simulink model "Tracking"  (R2017a)
settings: Solver=VariableStepAuto  StartTime=0.0  StopTime=0.5  RelTol=1e-3
undefined symbols (not defined in the file): magnitude
libraries: commfilt2 x24, simulink x16, dspmtrx3 x12, dspswit3 x8
(part 2 of 2)

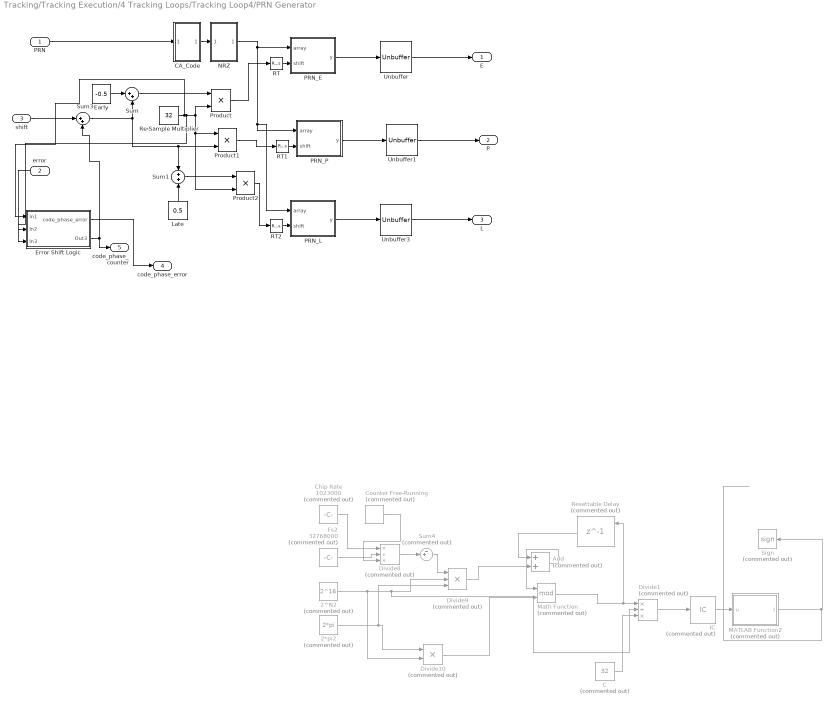
== system Tracking/Tracking Execution/4 Tracking Loops/Tracking Loop4/PRN Generator  ==
  PRN : Inport
  error : Inport  Port=2  SampleTime=0.001
  shift : Inport  Port=3
  2*pi2 : Constant  Commented=on  Value=2*pi
  2^N2 : Constant  Commented=on  Value=2^16
  Add : Sum  Commented=on
  C : Constant  Commented=on  Value=32
  "CA_Code " : Subsystem
  Chip Rate : Constant  Commented=on  Value=1023000
  Counter Free-Running : simulink/Sources/Counter Free-Running  Commented=on  NumBits=15  tsamp=1/32768000
  Divide1 : Product  Commented=on  Inputs=*/*
  Divide10 : Product  Commented=on
  Divide8 : Product  Commented=on  Inputs=*/*
  Divide9 : Product  Commented=on  Inputs=***
  Early : Constant  Value=-0.5
  Error Shift Logic : Subsystem
  Fs2 : Constant  Commented=on  Value=32768000
  IC : InitialCondition  Commented=on  Value=1023000
  Late : Constant  Value=0.5
  MATLAB Function2 : MATLAB Function  Commented=on  TreatAsAtomicUnit=on
  Math Function : Math  Commented=on  Operator=mod  SaturateOnIntegerOverflow=on
  NRZ : Subsystem
  PRN_E : MATLAB Function  TreatAsAtomicUnit=on  SystemSampleTime=0.001
  PRN_L : MATLAB Function  TreatAsAtomicUnit=on  SystemSampleTime=0.001
  PRN_P : MATLAB Function  TreatAsAtomicUnit=on  SystemSampleTime=0.001
  Product : Product
  Product1 : Product
  Product2 : Product
  RT : RateTransition  OutPortSampleTime=0.001
  RT1 : RateTransition  OutPortSampleTime=0.001
  RT2 : RateTransition  OutPortSampleTime=0.001
  Re-Sample Multiplier : Constant  Value=32
  Resettable Delay : Delay  Commented=on  DelayLength=1  ExternalReset=Rising  SampleTime=0.001
      settings: InputPortMap=u0,r5
  Sign : Signum  Commented=on
  Sum : Sum  Inputs=|++
  Sum1 : Sum
  Sum3 : Sum  Inputs=|++
  Sum4 : Sum  Commented=on  Inputs=-+|
  Unbuffer : Unbuffer
  Unbuffer1 : Unbuffer
  Unbuffer3 : Unbuffer
  E : Outport
  P : Outport  Port=2
  L : Outport  Port=3
  code_phase_error : Outport  Port=4
  code_phase_counter : Outport  Port=5
  wires:
  Product/1 -> RT/1
  PRN_E/1(y) -> Unbuffer/1
  Product2/1 -> RT2/1
  PRN_L/1(y) -> Unbuffer3/1
  Re-Sample Multiplier/1 -> Error Shift Logic/1(In1), Error Shift Logic/2(In2), Product1/1, Product2/2, Product/2
  PRN/1 -> "CA_Code "/1(In1)
  Unbuffer1/1 -> P/1
  Unbuffer3/1 -> L/1
  Early/1 -> Sum/1
  Sum/1 -> Product/1
  Sum3/1 -> Product1/2, Sum1/1, Sum/2
  Sum1/1 -> Product2/1
  PRN_P/1(y) -> Unbuffer1/1
  RT/1 -> PRN_E/2(shift)
  RT1/1 -> PRN_P/2(shift)
  RT2/1 -> PRN_L/2(shift)
  Late/1 -> Sum1/2
  "CA_Code "/1(Out1) -> NRZ/1(In1)
  Unbuffer/1 -> E/1
  NRZ/1(Out1) -> PRN_E/1(array), PRN_L/1(array), PRN_P/1(array)
  Product1/1 -> RT1/1
  MATLAB Function2/1(I) -> Sign/1
  Divide8/1 -> Sum4/2
  C/1 -> Divide1/3
  2^N2/1 -> Divide10/2, Divide1/2, Divide9/2
  Fs2/1 -> Divide8/2
  2*pi2/1 -> Divide9/3, Divide10/1
  Sum4/1 -> Divide9/1
  IC/1 -> MATLAB Function2/1(u)
  Divide10/1 -> Math Function/2
  Chip Rate/1 -> Divide8/1
  Resettable Delay/1 -> Add/1
  Divide1/1 -> IC/1
  Divide9/1 -> Add/2
  Counter Free-Running/1 -> Divide8/3
  Add/1 -> Math Function/1
  Math Function/1 -> Resettable Delay/1, Divide1/1
  shift/1 -> Sum3/1
  Error Shift Logic/2(Out3) -> code_phase_counter/1, Sum3/2
  error/1 -> Error Shift Logic/3(In3)
  Error Shift Logic/1(code_phase_error) -> code_phase_error/1

== system Tracking/Tracking Execution/4 Tracking Loops/Tracking Loop1/Carrier Filter/Subsystem ==
  BW : Constant  Value=50
  C1 : Subsystem
  C2 : Subsystem
  Constant1 : Constant  Value=8
  Constant2 : Constant  Value=4
  Constant4 : Constant
  Damping : Constant  Value=0.7
  K : Constant  Value=4
  T : Constant  Value=0.001
  Wn : Subsystem
  "K2 " : Outport
  K1 : Outport  Port=2
  wires:
  C1/1(Out1) -> K1/1
  Constant1/1 -> C1/1(In1), Wn/1(In1)
  BW/1 -> Wn/2(In2)
  Damping/1 -> C1/2(In2), C1/3(In3), Wn/3(In3), C2/3(In3), C2/2(In2)
  Constant2/1 -> C2/5(In5), C1/7(In7), C2/6(In6), C2/7(In7), C1/8(In8), Wn/4(In4)
  Constant4/1 -> Wn/5(In5)
  T/1 -> C1/4(In4), C1/5(In5), C1/6(In6), C2/4(In4)
  Wn/1(Out1) -> C1/10(In10), C2/8(In8), C1/9(In9)
  C2/1(Out1) -> "K2 "/1
  K/1 -> C1/11(In11), C2/1(In1)

== system Tracking/Tracking Execution/4 Tracking Loops/Tracking Loop1/PRN Generator /CA_Code  ==
  In1 : Inport
  CA_Code : MATLAB Function  TreatAsAtomicUnit=on  SystemSampleTime=0.001
  Constant1 : Constant  Value=32
  Constant2 : Constant
  MinMax : MinMax  Function=max  Inputs=2
  RT : RateTransition  OutPortSampleTime=0.001
  Reshape : Reshape  OutputDimensionality=Column vector (2-D)
  Out1 : Outport
  wires:
  In1/1 -> RT/1
  CA_Code/1(g) -> Reshape/1
  Constant1/1 -> CA_Code/2(fs)
  Reshape/1 -> Out1/1
  RT/1 -> MinMax/2
  MinMax/1 -> CA_Code/1(sv)
  Constant2/1 -> MinMax/1

== system Tracking/Tracking Execution/4 Tracking Loops/Tracking Loop1/PRN Generator /Error Shift Logic ==
  In1 : Inport
  In2 : Inport  Port=2
  In3 : Inport  Port=3
  Compare To Constant2 : simulink/Logic and Bit Operations/Compare To Constant  relop=>=  const=1  OutDataTypeStr=uint8
  Compare To Constant3 : simulink/Logic and Bit Operations/Compare To Constant  relop=<=  const=-1  OutDataTypeStr=uint8
  Counter : dspswit3/Counter  Direction=Up  CountEvent=Non-zero sample  CounterSize=User defined  MaxCount=2^16  InitialCount=0  Output=Count  HitValue=32  ResetInput=off  SamplesPerFrame=1  Ts=1  CntDtype=double  HitDtype=Logical
  Counter1 : dspswit3/Counter  Direction=Up  CountEvent=Non-zero sample  CounterSize=User defined  MaxCount=2^16  InitialCount=0  Output=Count  HitValue=32  ResetInput=on  SamplesPerFrame=1  Ts=1  CntDtype=double  HitDtype=Logical
  Divide : Product  Inputs=*/
  Product3 : Product
  RT3 : RateTransition  OutPortSampleTime=0.001
  RT4 : RateTransition  OutPortSampleTime=0.001
  Rounding Function : Rounding  Operator=round
  Sum2 : Sum  Inputs=-+
  Sum5 : Sum  Inputs=+-
  Sum6 : Sum  Inputs=+-
  Unit Delay : UnitDelay  SampleTime=0.001
  code_phase_error : Outport
  Out3 : Outport  Port=2
  wires:
  Sum2/1 -> Divide/1
  Counter1/1 -> Sum2/2
  In3/1 -> Product3/1
  Counter/1 -> Sum2/1
  Unit Delay/1 -> Sum6/2
  Sum6/1 -> Sum5/1, Rounding Function/1
  Rounding Function/1 -> Sum5/2, Compare To Constant3/1, Compare To Constant2/1
  Compare To Constant2/1 -> RT4/1
  Sum5/1 -> Unit Delay/1
  RT3/1 -> Counter1/1
  Compare To Constant3/1 -> RT3/1
  Divide/1 -> Out3/1, code_phase_error/1
  Product3/1 -> Sum6/1
  RT4/1 -> Counter/1
  In1/1 -> Divide/2
  In2/1 -> Product3/2

== system Tracking/Tracking Execution/4 Tracking Loops/Tracking Loop1/PRN Generator /NRZ ==
  In1 : Inport
  Constant5 : Constant  Value=2  SampleTime=-1
  Constant6 : Constant  Value=-1
  Product4 : Product
  Sum4 : Sum  Inputs=|++
  Out1 : Outport
  wires:
  Constant6/1 -> Sum4/1
  Sum4/1 -> Out1/1
  Product4/1 -> Sum4/2
  In1/1 -> Product4/2
  Constant5/1 -> Product4/1

== system Tracking/Tracking Execution/4 Tracking Loops/Tracking Loop2/Carrier Filter/Subsystem ==
  BW : Constant  Value=50
  C1 : Subsystem
  C2 : Subsystem
  Constant1 : Constant  Value=8
  Constant2 : Constant  Value=4
  Constant4 : Constant
  Damping : Constant  Value=0.7
  K : Constant  Value=4
  T : Constant  Value=0.001
  Wn : Subsystem
  "K2 " : Outport
  K1 : Outport  Port=2
  wires:
  C1/1(Out1) -> K1/1
  Constant1/1 -> C1/1(In1), Wn/1(In1)
  BW/1 -> Wn/2(In2)
  Damping/1 -> C1/2(In2), C1/3(In3), Wn/3(In3), C2/3(In3), C2/2(In2)
  Constant2/1 -> C2/5(In5), C1/7(In7), C2/6(In6), C2/7(In7), C1/8(In8), Wn/4(In4)
  Constant4/1 -> Wn/5(In5)
  T/1 -> C1/4(In4), C1/5(In5), C1/6(In6), C2/4(In4)
  Wn/1(Out1) -> C1/10(In10), C2/8(In8), C1/9(In9)
  C2/1(Out1) -> "K2 "/1
  K/1 -> C1/11(In11), C2/1(In1)

== system Tracking/Tracking Execution/4 Tracking Loops/Tracking Loop2/PRN Generator /CA_Code  ==
  In1 : Inport
  CA_Code : MATLAB Function  TreatAsAtomicUnit=on  SystemSampleTime=0.001
  Constant1 : Constant  Value=32
  Constant2 : Constant
  MinMax : MinMax  Function=max  Inputs=2
  RT : RateTransition  OutPortSampleTime=0.001
  Reshape : Reshape  OutputDimensionality=Column vector (2-D)
  Out1 : Outport
  wires:
  In1/1 -> RT/1
  CA_Code/1(g) -> Reshape/1
  Constant1/1 -> CA_Code/2(fs)
  Reshape/1 -> Out1/1
  RT/1 -> MinMax/2
  MinMax/1 -> CA_Code/1(sv)
  Constant2/1 -> MinMax/1

== system Tracking/Tracking Execution/4 Tracking Loops/Tracking Loop2/PRN Generator /Error Shift Logic ==
  In1 : Inport
  In2 : Inport  Port=2
  In3 : Inport  Port=3
  Compare To Constant2 : simulink/Logic and Bit Operations/Compare To Constant  relop=>=  const=1  OutDataTypeStr=uint8
  Compare To Constant3 : simulink/Logic and Bit Operations/Compare To Constant  relop=<=  const=-1  OutDataTypeStr=uint8
  Counter : dspswit3/Counter  Direction=Up  CountEvent=Non-zero sample  CounterSize=User defined  MaxCount=2^16  InitialCount=0  Output=Count  HitValue=32  ResetInput=off  SamplesPerFrame=1  Ts=1  CntDtype=double  HitDtype=Logical
  Counter1 : dspswit3/Counter  Direction=Up  CountEvent=Non-zero sample  CounterSize=User defined  MaxCount=2^16  InitialCount=0  Output=Count  HitValue=32  ResetInput=on  SamplesPerFrame=1  Ts=1  CntDtype=double  HitDtype=Logical
  Divide : Product  Inputs=*/
  Product3 : Product
  RT3 : RateTransition  OutPortSampleTime=0.001
  RT4 : RateTransition  OutPortSampleTime=0.001
  Rounding Function : Rounding  Operator=round
  Sum2 : Sum  Inputs=-+
  Sum5 : Sum  Inputs=+-
  Sum6 : Sum  Inputs=+-
  Unit Delay : UnitDelay  SampleTime=0.001
  code_phase_error : Outport
  Out3 : Outport  Port=2
  wires:
  Sum2/1 -> Divide/1
  Counter1/1 -> Sum2/2
  In3/1 -> Product3/1
  Counter/1 -> Sum2/1
  Unit Delay/1 -> Sum6/2
  Sum6/1 -> Sum5/1, Rounding Function/1
  Rounding Function/1 -> Sum5/2, Compare To Constant3/1, Compare To Constant2/1
  Compare To Constant2/1 -> RT4/1
  Sum5/1 -> Unit Delay/1
  RT3/1 -> Counter1/1
  Compare To Constant3/1 -> RT3/1
  Divide/1 -> Out3/1, code_phase_error/1
  Product3/1 -> Sum6/1
  RT4/1 -> Counter/1
  In1/1 -> Divide/2
  In2/1 -> Product3/2

== system Tracking/Tracking Execution/4 Tracking Loops/Tracking Loop2/PRN Generator /NRZ ==
  In1 : Inport
  Constant5 : Constant  Value=2  SampleTime=-1
  Constant6 : Constant  Value=-1
  Product4 : Product
  Sum4 : Sum  Inputs=|++
  Out1 : Outport
  wires:
  Constant6/1 -> Sum4/1
  Sum4/1 -> Out1/1
  Product4/1 -> Sum4/2
  In1/1 -> Product4/2
  Constant5/1 -> Product4/1

== system Tracking/Tracking Execution/4 Tracking Loops/Tracking Loop3/Carrier Filter/Subsystem ==
  BW : Constant  Value=50
  C1 : Subsystem
  C2 : Subsystem
  Constant1 : Constant  Value=8
  Constant2 : Constant  Value=4
  Constant4 : Constant
  Damping : Constant  Value=0.7
  K : Constant  Value=4
  T : Constant  Value=0.001
  Wn : Subsystem
  "K2 " : Outport
  K1 : Outport  Port=2
  wires:
  C1/1(Out1) -> K1/1
  Constant1/1 -> C1/1(In1), Wn/1(In1)
  BW/1 -> Wn/2(In2)
  Damping/1 -> C1/2(In2), C1/3(In3), Wn/3(In3), C2/3(In3), C2/2(In2)
  Constant2/1 -> C2/5(In5), C1/7(In7), C2/6(In6), C2/7(In7), C1/8(In8), Wn/4(In4)
  Constant4/1 -> Wn/5(In5)
  T/1 -> C1/4(In4), C1/5(In5), C1/6(In6), C2/4(In4)
  Wn/1(Out1) -> C1/10(In10), C2/8(In8), C1/9(In9)
  C2/1(Out1) -> "K2 "/1
  K/1 -> C1/11(In11), C2/1(In1)

== system Tracking/Tracking Execution/4 Tracking Loops/Tracking Loop3/PRN Generator /CA_Code  ==
  In1 : Inport
  CA_Code : MATLAB Function  TreatAsAtomicUnit=on  SystemSampleTime=0.001
  Constant1 : Constant  Value=32
  Constant2 : Constant
  MinMax : MinMax  Function=max  Inputs=2
  RT : RateTransition  OutPortSampleTime=0.001
  Reshape : Reshape  OutputDimensionality=Column vector (2-D)
  Out1 : Outport
  wires:
  In1/1 -> RT/1
  CA_Code/1(g) -> Reshape/1
  Constant1/1 -> CA_Code/2(fs)
  Reshape/1 -> Out1/1
  RT/1 -> MinMax/2
  MinMax/1 -> CA_Code/1(sv)
  Constant2/1 -> MinMax/1

== system Tracking/Tracking Execution/4 Tracking Loops/Tracking Loop3/PRN Generator /Error Shift Logic ==
  In1 : Inport
  In2 : Inport  Port=2
  In3 : Inport  Port=3
  Compare To Constant2 : simulink/Logic and Bit Operations/Compare To Constant  relop=>=  const=1  OutDataTypeStr=uint8
  Compare To Constant3 : simulink/Logic and Bit Operations/Compare To Constant  relop=<=  const=-1  OutDataTypeStr=uint8
  Counter : dspswit3/Counter  Direction=Up  CountEvent=Non-zero sample  CounterSize=User defined  MaxCount=2^16  InitialCount=0  Output=Count  HitValue=32  ResetInput=off  SamplesPerFrame=1  Ts=1  CntDtype=double  HitDtype=Logical
  Counter1 : dspswit3/Counter  Direction=Up  CountEvent=Non-zero sample  CounterSize=User defined  MaxCount=2^16  InitialCount=0  Output=Count  HitValue=32  ResetInput=on  SamplesPerFrame=1  Ts=1  CntDtype=double  HitDtype=Logical
  Divide : Product  Inputs=*/
  Product3 : Product
  RT3 : RateTransition  OutPortSampleTime=0.001
  RT4 : RateTransition  OutPortSampleTime=0.001
  Rounding Function : Rounding  Operator=round
  Sum2 : Sum  Inputs=-+
  Sum5 : Sum  Inputs=+-
  Sum6 : Sum  Inputs=+-
  Unit Delay : UnitDelay  SampleTime=0.001
  code_phase_error : Outport
  Out3 : Outport  Port=2
  wires:
  Sum2/1 -> Divide/1
  Counter1/1 -> Sum2/2
  In3/1 -> Product3/1
  Counter/1 -> Sum2/1
  Unit Delay/1 -> Sum6/2
  Sum6/1 -> Sum5/1, Rounding Function/1
  Rounding Function/1 -> Sum5/2, Compare To Constant3/1, Compare To Constant2/1
  Compare To Constant2/1 -> RT4/1
  Sum5/1 -> Unit Delay/1
  RT3/1 -> Counter1/1
  Compare To Constant3/1 -> RT3/1
  Divide/1 -> Out3/1, code_phase_error/1
  Product3/1 -> Sum6/1
  RT4/1 -> Counter/1
  In1/1 -> Divide/2
  In2/1 -> Product3/2

== system Tracking/Tracking Execution/4 Tracking Loops/Tracking Loop3/PRN Generator /NRZ ==
  In1 : Inport
  Constant5 : Constant  Value=2  SampleTime=-1
  Constant6 : Constant  Value=-1
  Product4 : Product
  Sum4 : Sum  Inputs=|++
  Out1 : Outport
  wires:
  Constant6/1 -> Sum4/1
  Sum4/1 -> Out1/1
  Product4/1 -> Sum4/2
  In1/1 -> Product4/2
  Constant5/1 -> Product4/1

== system Tracking/Tracking Execution/4 Tracking Loops/Tracking Loop4/Carrier Filter/Subsystem ==
  BW : Constant  Value=50
  C1 : Subsystem
  C2 : Subsystem
  Constant1 : Constant  Value=8
  Constant2 : Constant  Value=4
  Constant4 : Constant
  Damping : Constant  Value=0.7
  K : Constant  Value=4
  T : Constant  Value=0.001
  Wn : Subsystem
  "K2 " : Outport
  K1 : Outport  Port=2
  wires:
  C1/1(Out1) -> K1/1
  Constant1/1 -> C1/1(In1), Wn/1(In1)
  BW/1 -> Wn/2(In2)
  Damping/1 -> C1/2(In2), C1/3(In3), Wn/3(In3), C2/3(In3), C2/2(In2)
  Constant2/1 -> C2/5(In5), C1/7(In7), C2/6(In6), C2/7(In7), C1/8(In8), Wn/4(In4)
  Constant4/1 -> Wn/5(In5)
  T/1 -> C1/4(In4), C1/5(In5), C1/6(In6), C2/4(In4)
  Wn/1(Out1) -> C1/10(In10), C2/8(In8), C1/9(In9)
  C2/1(Out1) -> "K2 "/1
  K/1 -> C1/11(In11), C2/1(In1)

== system Tracking/Tracking Execution/4 Tracking Loops/Tracking Loop4/PRN Generator /CA_Code  ==
  In1 : Inport
  CA_Code : MATLAB Function  TreatAsAtomicUnit=on  SystemSampleTime=0.001
  Constant1 : Constant  Value=32
  Constant2 : Constant
  MinMax : MinMax  Function=max  Inputs=2
  RT : RateTransition  OutPortSampleTime=0.001
  Reshape : Reshape  OutputDimensionality=Column vector (2-D)
  Out1 : Outport
  wires:
  In1/1 -> RT/1
  CA_Code/1(g) -> Reshape/1
  Constant1/1 -> CA_Code/2(fs)
  Reshape/1 -> Out1/1
  RT/1 -> MinMax/2
  MinMax/1 -> CA_Code/1(sv)
  Constant2/1 -> MinMax/1

== system Tracking/Tracking Execution/4 Tracking Loops/Tracking Loop4/PRN Generator /Error Shift Logic ==
  In1 : Inport
  In2 : Inport  Port=2
  In3 : Inport  Port=3
  Compare To Constant2 : simulink/Logic and Bit Operations/Compare To Constant  relop=>=  const=1  OutDataTypeStr=uint8
  Compare To Constant3 : simulink/Logic and Bit Operations/Compare To Constant  relop=<=  const=-1  OutDataTypeStr=uint8
  Counter : dspswit3/Counter  Direction=Up  CountEvent=Non-zero sample  CounterSize=User defined  MaxCount=2^16  InitialCount=0  Output=Count  HitValue=32  ResetInput=off  SamplesPerFrame=1  Ts=1  CntDtype=double  HitDtype=Logical
  Counter1 : dspswit3/Counter  Direction=Up  CountEvent=Non-zero sample  CounterSize=User defined  MaxCount=2^16  InitialCount=0  Output=Count  HitValue=32  ResetInput=on  SamplesPerFrame=1  Ts=1  CntDtype=double  HitDtype=Logical
  Divide : Product  Inputs=*/
  Product3 : Product
  RT3 : RateTransition  OutPortSampleTime=0.001
  RT4 : RateTransition  OutPortSampleTime=0.001
  Rounding Function : Rounding  Operator=round
  Sum2 : Sum  Inputs=-+
  Sum5 : Sum  Inputs=+-
  Sum6 : Sum  Inputs=+-
  Unit Delay : UnitDelay  SampleTime=0.001
  code_phase_error : Outport
  Out3 : Outport  Port=2
  wires:
  Sum2/1 -> Divide/1
  Counter1/1 -> Sum2/2
  In3/1 -> Product3/1
  Counter/1 -> Sum2/1
  Unit Delay/1 -> Sum6/2
  Sum6/1 -> Sum5/1, Rounding Function/1
  Rounding Function/1 -> Sum5/2, Compare To Constant3/1, Compare To Constant2/1
  Compare To Constant2/1 -> RT4/1
  Sum5/1 -> Unit Delay/1
  RT3/1 -> Counter1/1
  Compare To Constant3/1 -> RT3/1
  Divide/1 -> Out3/1, code_phase_error/1
  Product3/1 -> Sum6/1
  RT4/1 -> Counter/1
  In1/1 -> Divide/2
  In2/1 -> Product3/2

== system Tracking/Tracking Execution/4 Tracking Loops/Tracking Loop4/PRN Generator /NRZ ==
  In1 : Inport
  Constant5 : Constant  Value=2  SampleTime=-1
  Constant6 : Constant  Value=-1
  Product4 : Product
  Sum4 : Sum  Inputs=|++
  Out1 : Outport
  wires:
  Constant6/1 -> Sum4/1
  Sum4/1 -> Out1/1
  Product4/1 -> Sum4/2
  In1/1 -> Product4/2
  Constant5/1 -> Product4/1

== system Tracking/Tracking Execution/4 Tracking Loops/Tracking Loop1/Carrier Filter/Subsystem/C1 ==
  In1 : Inport
  In2 : Inport  Port=2
  In3 : Inport  Port=3
  In4 : Inport  Port=4
  In5 : Inport  Port=5
  In6 : Inport  Port=6
  In7 : Inport  Port=7
  In8 : Inport  Port=8
  In9 : Inport  Port=9
  In10 : Inport  Port=10
  In11 : Inport  Port=11
  Add1 : Sum  Inputs=+++
  Gain 3 : Product  Inputs=***/
  Gain 4 : Product  Inputs=***
  Math Function3 : Math  Operator=square  SaturateOnIntegerOverflow=on
  Product3 : Product
  Product4 : Product  Inputs=4
  Out1 : Outport
  wires:
  In5/1 -> Product4/4
  In7/1 -> Add1/3
  Gain 3/1 -> Out1/1
  In9/1 -> Product4/3
  In4/1 -> Product3/1
  In8/1 -> Product4/1
  In2/1 -> Gain 4/1
  In11/1 -> Gain 3/1
  In10/1 -> Product3/2, Gain 4/2
  In1/1 -> Gain 3/3
  In6/1 -> Gain 4/3
  In3/1 -> Product4/2
  Add1/1 -> Gain 3/4
  Product4/1 -> Add1/2
  Gain 4/1 -> Gain 3/2
  Math Function3/1 -> Add1/1
  Product3/1 -> Math Function3/1

== system Tracking/Tracking Execution/4 Tracking Loops/Tracking Loop1/Carrier Filter/Subsystem/C2 ==
  In1 : Inport
  In2 : Inport  Port=2
  In3 : Inport  Port=3
  In4 : Inport  Port=4
  In5 : Inport  Port=5
  In6 : Inport  Port=6
  In7 : Inport  Port=7
  In8 : Inport  Port=8
  Add : Sum  Inputs=+++
  Gain 1 : Product  Inputs=***/
  Gain 2 : Product  Inputs=***
  Math Function : Math  Operator=square  SaturateOnIntegerOverflow=on
  Math Function1 : Math  Operator=square  SaturateOnIntegerOverflow=on
  Product1 : Product
  Product2 : Product  Inputs=4
  Out1 : Outport
  wires:
  Product1/1 -> Math Function1/1
  Math Function1/1 -> Add/1
  Add/1 -> Gain 1/4
  In2/1 -> Gain 2/1
  In5/1 -> Add/3
  In7/1 -> Product2/1
  In3/1 -> Product2/2
  In1/1 -> Gain 1/3
  In6/1 -> Gain 1/2
  Product2/1 -> Add/2
  Gain 1/1 -> Out1/1
  Math Function/1 -> Gain 1/1
  In8/1 -> Product1/1, Gain 2/2, Product2/3
  In4/1 -> Product1/2, Product2/4, Gain 2/3
  Gain 2/1 -> Math Function/1

== system Tracking/Tracking Execution/4 Tracking Loops/Tracking Loop1/Carrier Filter/Subsystem/Wn ==
  In1 : Inport
  In2 : Inport  Port=2
  In3 : Inport  Port=3
  In4 : Inport  Port=4
  In5 : Inport  Port=5
  Add : Sum
  Divide1 : Product  Inputs=***/
  Math Function : Math  Operator=square  SaturateOnIntegerOverflow=on
  Wn1 : Product
  Out1 : Outport
  wires:
  In4/1 -> Wn1/2
  Add/1 -> Divide1/4
  Wn1/1 -> Add/1
  In3/1 -> Divide1/3, Math Function/1
  In2/1 -> Divide1/2
  Math Function/1 -> Wn1/1
  Divide1/1 -> Out1/1
  In1/1 -> Divide1/1
  In5/1 -> Add/2

== system Tracking/Tracking Execution/4 Tracking Loops/Tracking Loop2/Carrier Filter/Subsystem/C1 ==
  In1 : Inport
  In2 : Inport  Port=2
  In3 : Inport  Port=3
  In4 : Inport  Port=4
  In5 : Inport  Port=5
  In6 : Inport  Port=6
  In7 : Inport  Port=7
  In8 : Inport  Port=8
  In9 : Inport  Port=9
  In10 : Inport  Port=10
  In11 : Inport  Port=11
  Add1 : Sum  Inputs=+++
  Gain 3 : Product  Inputs=***/
  Gain 4 : Product  Inputs=***
  Math Function3 : Math  Operator=square  SaturateOnIntegerOverflow=on
  Product3 : Product
  Product4 : Product  Inputs=4
  Out1 : Outport
  wires:
  In5/1 -> Product4/4
  In7/1 -> Add1/3
  Gain 3/1 -> Out1/1
  In9/1 -> Product4/3
  In4/1 -> Product3/1
  In8/1 -> Product4/1
  In2/1 -> Gain 4/1
  In11/1 -> Gain 3/1
  In10/1 -> Product3/2, Gain 4/2
  In1/1 -> Gain 3/3
  In6/1 -> Gain 4/3
  In3/1 -> Product4/2
  Add1/1 -> Gain 3/4
  Product4/1 -> Add1/2
  Gain 4/1 -> Gain 3/2
  Math Function3/1 -> Add1/1
  Product3/1 -> Math Function3/1

== system Tracking/Tracking Execution/4 Tracking Loops/Tracking Loop2/Carrier Filter/Subsystem/C2 ==
  In1 : Inport
  In2 : Inport  Port=2
  In3 : Inport  Port=3
  In4 : Inport  Port=4
  In5 : Inport  Port=5
  In6 : Inport  Port=6
  In7 : Inport  Port=7
  In8 : Inport  Port=8
  Add : Sum  Inputs=+++
  Gain 1 : Product  Inputs=***/
  Gain 2 : Product  Inputs=***
  Math Function : Math  Operator=square  SaturateOnIntegerOverflow=on
  Math Function1 : Math  Operator=square  SaturateOnIntegerOverflow=on
  Product1 : Product
  Product2 : Product  Inputs=4
  Out1 : Outport
  wires:
  Product1/1 -> Math Function1/1
  Math Function1/1 -> Add/1
  Add/1 -> Gain 1/4
  In2/1 -> Gain 2/1
  In5/1 -> Add/3
  In7/1 -> Product2/1
  In3/1 -> Product2/2
  In1/1 -> Gain 1/3
  In6/1 -> Gain 1/2
  Product2/1 -> Add/2
  Gain 1/1 -> Out1/1
  Math Function/1 -> Gain 1/1
  In8/1 -> Product1/1, Gain 2/2, Product2/3
  In4/1 -> Product1/2, Product2/4, Gain 2/3
  Gain 2/1 -> Math Function/1

== system Tracking/Tracking Execution/4 Tracking Loops/Tracking Loop2/Carrier Filter/Subsystem/Wn ==
  In1 : Inport
  In2 : Inport  Port=2
  In3 : Inport  Port=3
  In4 : Inport  Port=4
  In5 : Inport  Port=5
  Add : Sum
  Divide1 : Product  Inputs=***/
  Math Function : Math  Operator=square  SaturateOnIntegerOverflow=on
  Wn1 : Product
  Out1 : Outport
  wires:
  In4/1 -> Wn1/2
  Add/1 -> Divide1/4
  Wn1/1 -> Add/1
  In3/1 -> Divide1/3, Math Function/1
  In2/1 -> Divide1/2
  Math Function/1 -> Wn1/1
  Divide1/1 -> Out1/1
  In1/1 -> Divide1/1
  In5/1 -> Add/2

== system Tracking/Tracking Execution/4 Tracking Loops/Tracking Loop3/Carrier Filter/Subsystem/C1 ==
  In1 : Inport
  In2 : Inport  Port=2
  In3 : Inport  Port=3
  In4 : Inport  Port=4
  In5 : Inport  Port=5
  In6 : Inport  Port=6
  In7 : Inport  Port=7
  In8 : Inport  Port=8
  In9 : Inport  Port=9
  In10 : Inport  Port=10
  In11 : Inport  Port=11
  Add1 : Sum  Inputs=+++
  Gain 3 : Product  Inputs=***/
  Gain 4 : Product  Inputs=***
  Math Function3 : Math  Operator=square  SaturateOnIntegerOverflow=on
  Product3 : Product
  Product4 : Product  Inputs=4
  Out1 : Outport
  wires:
  In5/1 -> Product4/4
  In7/1 -> Add1/3
  Gain 3/1 -> Out1/1
  In9/1 -> Product4/3
  In4/1 -> Product3/1
  In8/1 -> Product4/1
  In2/1 -> Gain 4/1
  In11/1 -> Gain 3/1
  In10/1 -> Product3/2, Gain 4/2
  In1/1 -> Gain 3/3
  In6/1 -> Gain 4/3
  In3/1 -> Product4/2
  Add1/1 -> Gain 3/4
  Product4/1 -> Add1/2
  Gain 4/1 -> Gain 3/2
  Math Function3/1 -> Add1/1
  Product3/1 -> Math Function3/1

== system Tracking/Tracking Execution/4 Tracking Loops/Tracking Loop3/Carrier Filter/Subsystem/C2 ==
  In1 : Inport
  In2 : Inport  Port=2
  In3 : Inport  Port=3
  In4 : Inport  Port=4
  In5 : Inport  Port=5
  In6 : Inport  Port=6
  In7 : Inport  Port=7
  In8 : Inport  Port=8
  Add : Sum  Inputs=+++
  Gain 1 : Product  Inputs=***/
  Gain 2 : Product  Inputs=***
  Math Function : Math  Operator=square  SaturateOnIntegerOverflow=on
  Math Function1 : Math  Operator=square  SaturateOnIntegerOverflow=on
  Product1 : Product
  Product2 : Product  Inputs=4
  Out1 : Outport
  wires:
  Product1/1 -> Math Function1/1
  Math Function1/1 -> Add/1
  Add/1 -> Gain 1/4
  In2/1 -> Gain 2/1
  In5/1 -> Add/3
  In7/1 -> Product2/1
  In3/1 -> Product2/2
  In1/1 -> Gain 1/3
  In6/1 -> Gain 1/2
  Product2/1 -> Add/2
  Gain 1/1 -> Out1/1
  Math Function/1 -> Gain 1/1
  In8/1 -> Product1/1, Gain 2/2, Product2/3
  In4/1 -> Product1/2, Product2/4, Gain 2/3
  Gain 2/1 -> Math Function/1

== system Tracking/Tracking Execution/4 Tracking Loops/Tracking Loop3/Carrier Filter/Subsystem/Wn ==
  In1 : Inport
  In2 : Inport  Port=2
  In3 : Inport  Port=3
  In4 : Inport  Port=4
  In5 : Inport  Port=5
  Add : Sum
  Divide1 : Product  Inputs=***/
  Math Function : Math  Operator=square  SaturateOnIntegerOverflow=on
  Wn1 : Product
  Out1 : Outport
  wires:
  In4/1 -> Wn1/2
  Add/1 -> Divide1/4
  Wn1/1 -> Add/1
  In3/1 -> Divide1/3, Math Function/1
  In2/1 -> Divide1/2
  Math Function/1 -> Wn1/1
  Divide1/1 -> Out1/1
  In1/1 -> Divide1/1
  In5/1 -> Add/2

== system Tracking/Tracking Execution/4 Tracking Loops/Tracking Loop4/Carrier Filter/Subsystem/C1 ==
  In1 : Inport
  In2 : Inport  Port=2
  In3 : Inport  Port=3
  In4 : Inport  Port=4
  In5 : Inport  Port=5
  In6 : Inport  Port=6
  In7 : Inport  Port=7
  In8 : Inport  Port=8
  In9 : Inport  Port=9
  In10 : Inport  Port=10
  In11 : Inport  Port=11
  Add1 : Sum  Inputs=+++
  Gain 3 : Product  Inputs=***/
  Gain 4 : Product  Inputs=***
  Math Function3 : Math  Operator=square  SaturateOnIntegerOverflow=on
  Product3 : Product
  Product4 : Product  Inputs=4
  Out1 : Outport
  wires:
  In5/1 -> Product4/4
  In7/1 -> Add1/3
  Gain 3/1 -> Out1/1
  In9/1 -> Product4/3
  In4/1 -> Product3/1
  In8/1 -> Product4/1
  In2/1 -> Gain 4/1
  In11/1 -> Gain 3/1
  In10/1 -> Product3/2, Gain 4/2
  In1/1 -> Gain 3/3
  In6/1 -> Gain 4/3
  In3/1 -> Product4/2
  Add1/1 -> Gain 3/4
  Product4/1 -> Add1/2
  Gain 4/1 -> Gain 3/2
  Math Function3/1 -> Add1/1
  Product3/1 -> Math Function3/1

== system Tracking/Tracking Execution/4 Tracking Loops/Tracking Loop4/Carrier Filter/Subsystem/C2 ==
  In1 : Inport
  In2 : Inport  Port=2
  In3 : Inport  Port=3
  In4 : Inport  Port=4
  In5 : Inport  Port=5
  In6 : Inport  Port=6
  In7 : Inport  Port=7
  In8 : Inport  Port=8
  Add : Sum  Inputs=+++
  Gain 1 : Product  Inputs=***/
  Gain 2 : Product  Inputs=***
  Math Function : Math  Operator=square  SaturateOnIntegerOverflow=on
  Math Function1 : Math  Operator=square  SaturateOnIntegerOverflow=on
  Product1 : Product
  Product2 : Product  Inputs=4
  Out1 : Outport
  wires:
  Product1/1 -> Math Function1/1
  Math Function1/1 -> Add/1
  Add/1 -> Gain 1/4
  In2/1 -> Gain 2/1
  In5/1 -> Add/3
  In7/1 -> Product2/1
  In3/1 -> Product2/2
  In1/1 -> Gain 1/3
  In6/1 -> Gain 1/2
  Product2/1 -> Add/2
  Gain 1/1 -> Out1/1
  Math Function/1 -> Gain 1/1
  In8/1 -> Product1/1, Gain 2/2, Product2/3
  In4/1 -> Product1/2, Product2/4, Gain 2/3
  Gain 2/1 -> Math Function/1

== system Tracking/Tracking Execution/4 Tracking Loops/Tracking Loop4/Carrier Filter/Subsystem/Wn ==
  In1 : Inport
  In2 : Inport  Port=2
  In3 : Inport  Port=3
  In4 : Inport  Port=4
  In5 : Inport  Port=5
  Add : Sum
  Divide1 : Product  Inputs=***/
  Math Function : Math  Operator=square  SaturateOnIntegerOverflow=on
  Wn1 : Product
  Out1 : Outport
  wires:
  In4/1 -> Wn1/2
  Add/1 -> Divide1/4
  Wn1/1 -> Add/1
  In3/1 -> Divide1/3, Math Function/1
  In2/1 -> Divide1/2
  Math Function/1 -> Wn1/1
  Divide1/1 -> Out1/1
  In1/1 -> Divide1/1
  In5/1 -> Add/2

== matlab function Tracking/Tracking Execution/4 Tracking Loops/Tracking Loop1/PRN Generator /CA_Code /CA_Code ==
  data: sv input; g output; fs input
function g=CAcode(sv,fs)
coder.extrinsic('warning')
% function G=CACODE(SV,FS) 
% Generates 1023 length C/A Codes for GPS PRNs 1-37
%
% 
% g: nx1023 matrix- with each PRN in each row with symbols 1 and 0
% sv: a row or column vector of the SV's to be generated
% 	 valid entries are 1 to 37
% fs: optional number of samples per chip (defaults to 1), fractional samples allowed, must be 1 or greater.
%
% For multiple samples per chip, function is a zero order hold. 
%
%
% For example to generate the C/A codes for PRN 6 and PRN 12 use:
% g=cacode([6 12]),
% and to generate the C/A codes for PRN 6 and PRN 12 at 5 MHz use
% g=cacode([6 12],5/1.023)
% 
%
% For more information refer to the "GPS SPS Signal Specification"
% http://www.navcen.uscg.gov/pubs/gps/sigspec/default.htm
%
% Dan Boschen 12-30-2007
% boschen@loglin.com

% Revision History
% rev 1.0 Dan Boschen 4-15-2007  Initial Release
%
% rev 1.1 Dan Boschen 7-15-2007  Corrected error with taps for PRN30, should be [2,7] was 
% 					incorrect as [1 7]. Thank you Jadah Zak for finding this.
%
%
% rev 1.2 Dan Boschen 12-26-2007 Fixed column index error when ceil ~ L 
%				Thank you Jared Meadows for finding this.
%
% rev 1.3 Dan Boschen 12-30-2007 Changed comment "first order hold" to
% "zero order hold".
%
% rev 1.4 Dan Boschen 6-1-2010   Updated email address in comments



if nargin<2
	fs=1;
end


if (max(sv)>37) || (min(sv)<1) || (min(size(sv))~=1)
	error('sv must be a row or column vector with integers between 1 and 37\n')
end

if fs<1
	error('fs must be 1 or greater\n')
end	

% force integers
testint=round(sv)-sv;
if testint ~= 0 
	warning('non-integer value entered for sv, rounding to closest integer\n');
	sv = round(sv);
end


% table of C/A Code Tap Selection (sets delay for G2 generator)
tap=[2 6;
    3 7;
    4 8;
    5 9;
    1 9;
    2 10;
    1 8;
    2 9;
    3 10;
    2 3;
    3 4;
    5 6;
    6 7;
    7 8;
    8 9;
    9 10;
    1 4;
    2 5;
    3 6;
    4 7;
    5 8;
    6 9;
    1 3;
    4 6;
    5 7;
    6 8;
    7 9;
    8 10;
    1 6;
    2 7;
    3 8;
    4 9
    5 10
    4 10
    1 7
    2 8
    4 10];

% G1 LFSR: x^10+x^3+1
s=[0 0 1 0 0 0 0 0 0 1];
n=length(s);
g1=ones(1,n);	%initialization vector for G1

%g=ones(1,38192);
%g2=ones(1,38192);
%gfs=ones(1,38192);

g=ones(1,65536/2);
g2=ones(1,65536/2);
gfs=ones(1,65536/2);

L=2^n-1;

% G2j LFSR: x^10+x^9+x^8+x^6+x^3+x^2+1
t=[0 1 1 0 0 1 0 1 1 1];
q=ones(1,n);	%initialization vector for G2

% generate C/A Code sequences:
tap_sel=tap(sv,:);
for inc=1:L
    g2(:,inc)=mod(sum(q(tap_sel),2),2);
    g(:,inc)=mod(g1(n)+g2(:,inc),2);
   g1=[mod(sum(g1.*s),2) g1(1:n-1)];
   q=[mod(sum(q.*t),2) q(1:n-1)];
end

%upsample to desired rate
if fs~=1
	%fractional upsampling with zero order hold
	index=0;
	for cnt = 1/fs:1/fs:L
		index=index+1;
		if ceil(cnt) > L   %traps a floating point error in index
			gfs(:,index)=g(:,L);
		else
			gfs(:,index)=g(:,ceil(cnt));
		end
	end 
	g=gfs;
end

== matlab function Tracking/MATLAB Function ==
  data: y output
function y = fcn()

%FORMAT: [SATELLITE #1 Parameters, ... ,SATELLITE #4 parameters]
%y =[0 (SV#) (frequency) (code phase);... ; 0 (SV#) (frequency) (code phase);]  
y = [0 1 9207000 0; 0 2 9207000 100;0 3 9207000 512;0 4 9207000 800];

== matlab function Tracking/Tracking Execution/4 Tracking Loops/Tracking Loop1/Oscillator/MATLAB Function2 ==
  data: u input; I output; Q output
function [I,Q]= fcn(u)

I = cos(u);
Q = sin(u);

== matlab function Tracking/Tracking Execution/4 Tracking Loops/Tracking Loop1/PRN Generator /MATLAB Function2 ==
  data: u input; I output
function I = fcn(u)

I = cos(u);

== matlab function Tracking/Tracking Execution/4 Tracking Loops/Tracking Loop1/PRN Generator /PRN_E ==
  data: array input; y output; shift input
function y = fcn(array, shift)

y = circshift(array, shift);

== matlab function Tracking/Tracking Execution/4 Tracking Loops/Tracking Loop1/PRN Generator /PRN_L ==
  data: array input; y output; shift input
function y = fcn(array, shift)

y = circshift(array, shift);

== matlab function Tracking/Tracking Execution/4 Tracking Loops/Tracking Loop2/Oscillator/MATLAB Function2 ==
  data: u input; I output; Q output
function [I,Q]= fcn(u)

I = cos(u);
Q = sin(u);

== matlab function Tracking/Tracking Execution/4 Tracking Loops/Tracking Loop2/PRN Generator /CA_Code /CA_Code ==
  data: sv input; g output; fs input
function g=CAcode(sv,fs)
coder.extrinsic('warning')
% function G=CACODE(SV,FS) 
% Generates 1023 length C/A Codes for GPS PRNs 1-37
%
% 
% g: nx1023 matrix- with each PRN in each row with symbols 1 and 0
% sv: a row or column vector of the SV's to be generated
% 	 valid entries are 1 to 37
% fs: optional number of samples per chip (defaults to 1), fractional samples allowed, must be 1 or greater.
%
% For multiple samples per chip, function is a zero order hold. 
%
%
% For example to generate the C/A codes for PRN 6 and PRN 12 use:
% g=cacode([6 12]),
% and to generate the C/A codes for PRN 6 and PRN 12 at 5 MHz use
% g=cacode([6 12],5/1.023)
% 
%
% For more information refer to the "GPS SPS Signal Specification"
% http://www.navcen.uscg.gov/pubs/gps/sigspec/default.htm
%
% Dan Boschen 12-30-2007
% boschen@loglin.com

% Revision History
% rev 1.0 Dan Boschen 4-15-2007  Initial Release
%
% rev 1.1 Dan Boschen 7-15-2007  Corrected error with taps for PRN30, should be [2,7] was 
% 					incorrect as [1 7]. Thank you Jadah Zak for finding this.
%
%
% rev 1.2 Dan Boschen 12-26-2007 Fixed column index error when ceil ~ L 
%				Thank you Jared Meadows for finding this.
%
% rev 1.3 Dan Boschen 12-30-2007 Changed comment "first order hold" to
% "zero order hold".
%
% rev 1.4 Dan Boschen 6-1-2010   Updated email address in comments



if nargin<2
	fs=1;
end


if (max(sv)>37) || (min(sv)<1) || (min(size(sv))~=1)
	error('sv must be a row or column vector with integers between 1 and 37\n')
end

if fs<1
	error('fs must be 1 or greater\n')
end	

% force integers
testint=round(sv)-sv;
if testint ~= 0 
	warning('non-integer value entered for sv, rounding to closest integer\n');
	sv = round(sv);
end


% table of C/A Code Tap Selection (sets delay for G2 generator)
tap=[2 6;
    3 7;
    4 8;
    5 9;
    1 9;
    2 10;
    1 8;
    2 9;
    3 10;
    2 3;
    3 4;
    5 6;
    6 7;
    7 8;
    8 9;
    9 10;
    1 4;
    2 5;
    3 6;
    4 7;
    5 8;
    6 9;
    1 3;
    4 6;
    5 7;
    6 8;
    7 9;
    8 10;
    1 6;
    2 7;
    3 8;
    4 9
    5 10
    4 10
    1 7
    2 8
    4 10];

% G1 LFSR: x^10+x^3+1
s=[0 0 1 0 0 0 0 0 0 1];
n=length(s);
g1=ones(1,n);	%initialization vector for G1

%g=ones(1,38192);
%g2=ones(1,38192);
%gfs=ones(1,38192);

g=ones(1,65536/2);
g2=ones(1,65536/2);
gfs=ones(1,65536/2);

L=2^n-1;

% G2j LFSR: x^10+x^9+x^8+x^6+x^3+x^2+1
t=[0 1 1 0 0 1 0 1 1 1];
q=ones(1,n);	%initialization vector for G2

% generate C/A Code sequences:
tap_sel=tap(sv,:);
for inc=1:L
    g2(:,inc)=mod(sum(q(tap_sel),2),2);
    g(:,inc)=mod(g1(n)+g2(:,inc),2);
   g1=[mod(sum(g1.*s),2) g1(1:n-1)];
   q=[mod(sum(q.*t),2) q(1:n-1)];
end

%upsample to desired rate
if fs~=1
	%fractional upsampling with zero order hold
	index=0;
	for cnt = 1/fs:1/fs:L
		index=index+1;
		if ceil(cnt) > L   %traps a floating point error in index
			gfs(:,index)=g(:,L);
		else
			gfs(:,index)=g(:,ceil(cnt));
		end
	end 
	g=gfs;
end

== matlab function Tracking/Tracking Execution/4 Tracking Loops/Tracking Loop2/PRN Generator /MATLAB Function2 ==
  data: u input; I output
function I = fcn(u)

I = cos(u);

== matlab function Tracking/Tracking Execution/4 Tracking Loops/Tracking Loop2/PRN Generator /PRN_E ==
  data: array input; y output; shift input
function y = fcn(array, shift)

y = circshift(array, shift);

== matlab function Tracking/Tracking Execution/4 Tracking Loops/Tracking Loop1/PRN Generator /PRN_P ==
  data: array input; y output size=32768; shift input
function y = fcn(array, shift)

y = circshift(array, shift);

== matlab function Tracking/Tracking Execution/4 Tracking Loops/Tracking Loop3/PRN Generator /CA_Code /CA_Code ==
  data: sv input; g output; fs input
function g=CAcode(sv,fs)
coder.extrinsic('warning')
% function G=CACODE(SV,FS) 
% Generates 1023 length C/A Codes for GPS PRNs 1-37
%
% 
% g: nx1023 matrix- with each PRN in each row with symbols 1 and 0
% sv: a row or column vector of the SV's to be generated
% 	 valid entries are 1 to 37
% fs: optional number of samples per chip (defaults to 1), fractional samples allowed, must be 1 or greater.
%
% For multiple samples per chip, function is a zero order hold. 
%
%
% For example to generate the C/A codes for PRN 6 and PRN 12 use:
% g=cacode([6 12]),
% and to generate the C/A codes for PRN 6 and PRN 12 at 5 MHz use
% g=cacode([6 12],5/1.023)
% 
%
% For more information refer to the "GPS SPS Signal Specification"
% http://www.navcen.uscg.gov/pubs/gps/sigspec/default.htm
%
% Dan Boschen 12-30-2007
% boschen@loglin.com

% Revision History
% rev 1.0 Dan Boschen 4-15-2007  Initial Release
%
% rev 1.1 Dan Boschen 7-15-2007  Corrected error with taps for PRN30, should be [2,7] was 
% 					incorrect as [1 7]. Thank you Jadah Zak for finding this.
%
%
% rev 1.2 Dan Boschen 12-26-2007 Fixed column index error when ceil ~ L 
%				Thank you Jared Meadows for finding this.
%
% rev 1.3 Dan Boschen 12-30-2007 Changed comment "first order hold" to
% "zero order hold".
%
% rev 1.4 Dan Boschen 6-1-2010   Updated email address in comments



if nargin<2
	fs=1;
end


if (max(sv)>37) || (min(sv)<1) || (min(size(sv))~=1)
	error('sv must be a row or column vector with integers between 1 and 37\n')
end

if fs<1
	error('fs must be 1 or greater\n')
end	

% force integers
testint=round(sv)-sv;
if testint ~= 0 
	warning('non-integer value entered for sv, rounding to closest integer\n');
	sv = round(sv);
end


% table of C/A Code Tap Selection (sets delay for G2 generator)
tap=[2 6;
    3 7;
    4 8;
    5 9;
    1 9;
    2 10;
    1 8;
    2 9;
    3 10;
    2 3;
    3 4;
    5 6;
    6 7;
    7 8;
    8 9;
    9 10;
    1 4;
    2 5;
    3 6;
    4 7;
    5 8;
    6 9;
    1 3;
    4 6;
    5 7;
    6 8;
    7 9;
    8 10;
    1 6;
    2 7;
    3 8;
    4 9
    5 10
    4 10
    1 7
    2 8
    4 10];

% G1 LFSR: x^10+x^3+1
s=[0 0 1 0 0 0 0 0 0 1];
n=length(s);
g1=ones(1,n);	%initialization vector for G1

%g=ones(1,38192);
%g2=ones(1,38192);
%gfs=ones(1,38192);

g=ones(1,65536/2);
g2=ones(1,65536/2);
gfs=ones(1,65536/2);

L=2^n-1;

% G2j LFSR: x^10+x^9+x^8+x^6+x^3+x^2+1
t=[0 1 1 0 0 1 0 1 1 1];
q=ones(1,n);	%initialization vector for G2

% generate C/A Code sequences:
tap_sel=tap(sv,:);
for inc=1:L
    g2(:,inc)=mod(sum(q(tap_sel),2),2);
    g(:,inc)=mod(g1(n)+g2(:,inc),2);
   g1=[mod(sum(g1.*s),2) g1(1:n-1)];
   q=[mod(sum(q.*t),2) q(1:n-1)];
end

%upsample to desired rate
if fs~=1
	%fractional upsampling with zero order hold
	index=0;
	for cnt = 1/fs:1/fs:L
		index=index+1;
		if ceil(cnt) > L   %traps a floating point error in index
			gfs(:,index)=g(:,L);
		else
			gfs(:,index)=g(:,ceil(cnt));
		end
	end 
	g=gfs;
end

== matlab function Tracking/Tracking Execution/4 Tracking Loops/Tracking Loop3/Oscillator/MATLAB Function2 ==
  data: u input; I output; Q output
function [I,Q]= fcn(u)

I = cos(u);
Q = sin(u);

== matlab function Tracking/Tracking Execution/4 Tracking Loops/Tracking Loop2/PRN Generator /PRN_L ==
  data: array input; y output; shift input
function y = fcn(array, shift)

y = circshift(array, shift);

== matlab function Tracking/Tracking Execution/4 Tracking Loops/Tracking Loop3/PRN Generator /MATLAB Function2 ==
  data: u input; I output
function I = fcn(u)

I = cos(u);

== matlab function Tracking/Tracking Execution/4 Tracking Loops/Tracking Loop4/Oscillator/MATLAB Function2 ==
  data: u input; I output; Q output
function [I,Q]= fcn(u)

I = cos(u);
Q = sin(u);

== matlab function Tracking/Tracking Execution/4 Tracking Loops/Tracking Loop4/PRN Generator /CA_Code /CA_Code ==
  data: sv input; g output; fs input
function g=CAcode(sv,fs)
coder.extrinsic('warning')
% function G=CACODE(SV,FS) 
% Generates 1023 length C/A Codes for GPS PRNs 1-37
%
% 
% g: nx1023 matrix- with each PRN in each row with symbols 1 and 0
% sv: a row or column vector of the SV's to be generated
% 	 valid entries are 1 to 37
% fs: optional number of samples per chip (defaults to 1), fractional samples allowed, must be 1 or greater.
%
% For multiple samples per chip, function is a zero order hold. 
%
%
% For example to generate the C/A codes for PRN 6 and PRN 12 use:
% g=cacode([6 12]),
% and to generate the C/A codes for PRN 6 and PRN 12 at 5 MHz use
% g=cacode([6 12],5/1.023)
% 
%
% For more information refer to the "GPS SPS Signal Specification"
% http://www.navcen.uscg.gov/pubs/gps/sigspec/default.htm
%
% Dan Boschen 12-30-2007
% boschen@loglin.com

% Revision History
% rev 1.0 Dan Boschen 4-15-2007  Initial Release
%
% rev 1.1 Dan Boschen 7-15-2007  Corrected error with taps for PRN30, should be [2,7] was 
% 					incorrect as [1 7]. Thank you Jadah Zak for finding this.
%
%
% rev 1.2 Dan Boschen 12-26-2007 Fixed column index error when ceil ~ L 
%				Thank you Jared Meadows for finding this.
%
% rev 1.3 Dan Boschen 12-30-2007 Changed comment "first order hold" to
% "zero order hold".
%
% rev 1.4 Dan Boschen 6-1-2010   Updated email address in comments



if nargin<2
	fs=1;
end


if (max(sv)>37) || (min(sv)<1) || (min(size(sv))~=1)
	error('sv must be a row or column vector with integers between 1 and 37\n')
end

if fs<1
	error('fs must be 1 or greater\n')
end	

% force integers
testint=round(sv)-sv;
if testint ~= 0 
	warning('non-integer value entered for sv, rounding to closest integer\n');
	sv = round(sv);
end


% table of C/A Code Tap Selection (sets delay for G2 generator)
tap=[2 6;
    3 7;
    4 8;
    5 9;
    1 9;
    2 10;
    1 8;
    2 9;
    3 10;
    2 3;
    3 4;
    5 6;
    6 7;
    7 8;
    8 9;
    9 10;
    1 4;
    2 5;
    3 6;
    4 7;
    5 8;
    6 9;
    1 3;
    4 6;
    5 7;
    6 8;
    7 9;
    8 10;
    1 6;
    2 7;
    3 8;
    4 9
    5 10
    4 10
    1 7
    2 8
    4 10];

% G1 LFSR: x^10+x^3+1
s=[0 0 1 0 0 0 0 0 0 1];
n=length(s);
g1=ones(1,n);	%initialization vector for G1

%g=ones(1,38192);
%g2=ones(1,38192);
%gfs=ones(1,38192);

g=ones(1,65536/2);
g2=ones(1,65536/2);
gfs=ones(1,65536/2);

L=2^n-1;

% G2j LFSR: x^10+x^9+x^8+x^6+x^3+x^2+1
t=[0 1 1 0 0 1 0 1 1 1];
q=ones(1,n);	%initialization vector for G2

% generate C/A Code sequences:
tap_sel=tap(sv,:);
for inc=1:L
    g2(:,inc)=mod(sum(q(tap_sel),2),2);
    g(:,inc)=mod(g1(n)+g2(:,inc),2);
   g1=[mod(sum(g1.*s),2) g1(1:n-1)];
   q=[mod(sum(q.*t),2) q(1:n-1)];
end

%upsample to desired rate
if fs~=1
	%fractional upsampling with zero order hold
	index=0;
	for cnt = 1/fs:1/fs:L
		index=index+1;
		if ceil(cnt) > L   %traps a floating point error in index
			gfs(:,index)=g(:,L);
		else
			gfs(:,index)=g(:,ceil(cnt));
		end
	end 
	g=gfs;
end

== matlab function Tracking/Tracking Execution/4 Tracking Loops/Tracking Loop4/PRN Generator /MATLAB Function2 ==
  data: u input; I output
function I = fcn(u)

I = cos(u);

== matlab function Tracking/Tracking Execution/4 Tracking Loops/Tracking Loop2/PRN Generator /PRN_P ==
  data: array input; y output size=32768; shift input
function y = fcn(array, shift)

y = circshift(array, shift);

== matlab function Tracking/Tracking Execution/4 Tracking Loops/Tracking Loop3/PRN Generator /PRN_E ==
  data: array input; y output; shift input
function y = fcn(array, shift)

y = circshift(array, shift);

== matlab function Tracking/Tracking Execution/4 Tracking Loops/Tracking Loop4/PRN Generator /PRN_E ==
  data: array input; y output; shift input
function y = fcn(array, shift)

y = circshift(array, shift);

== matlab function Tracking/Tracking Execution/4 Tracking Loops/Tracking Loop3/PRN Generator /PRN_L ==
  data: array input; y output; shift input
function y = fcn(array, shift)

y = circshift(array, shift);

== matlab function Tracking/Tracking Execution/4 Tracking Loops/Tracking Loop3/PRN Generator /PRN_P ==
  data: array input; y output size=32768; shift input
function y = fcn(array, shift)

y = circshift(array, shift);

== matlab function Tracking/Tracking Execution/4 Tracking Loops/Tracking Loop4/PRN Generator /PRN_L ==
  data: array input; y output; shift input
function y = fcn(array, shift)

y = circshift(array, shift);

== matlab function Tracking/Tracking Execution/4 Tracking Loops/Tracking Loop4/PRN Generator /PRN_P ==
  data: array input; y output size=32768; shift input
function y = fcn(array, shift)

y = circshift(array, shift);
